simulink model "SeatMdSwtchArbt"  (R2018b)
settings: Solver=FixedStepDiscrete  StartTime=0.0  StopTime=10.0  FixedStep=0.01  RelTol=1e-3
undefined symbols (not defined in the file or in its folder): PosRclRspStat1
libraries: SeatMdSwtchArbt_Lib x35
(part 1 of 2)
settings Model: Creator=su3dcu  LastModifiedBy=su3dcu
settings DataIOCC: SaveFormat=StructureWithTime  ReturnWorkspaceOutputs=on
settings OptimizationCC: DefaultParameterBehavior=Inlined  EnhancedBackFolding=on  PassReuseOutputArgsAs=Individual arguments  ZeroExternalMemoryAtStartup=off  ZeroInternalMemoryAtStartup=off  OptimizeBlockOrder=speed  DifferentSizesBufferReuse=on  OptimizationCustomize=off
settings DebuggingCC: ParameterTunabilityLossMsg=error
settings HardwareCC: ProdBitPerPointer=32  ProdBitPerSizeT=32  ProdBitPerPtrDiffT=32  ProdLargestAtomicFloat=None  ProdWordSize=32  ProdHWDeviceType=Renesas->RH850
settings ModelReferenceCC: ModelReferenceNumInstancesAllowed=Single
settings SFSimCC: SimCustomHeaderCode="#include\"Rte_Type.h\""  MATLABDynamicMemAlloc=off
settings RTWCC: SystemTargetFile=autosar.tlc  GenCodeOnly=on  TemplateMakefile=ert_default_tmf  Description=AUTOSAR  GenerateReport=on  IncludeHyperlinkInReport=on  LaunchReport=on  CodeExecutionProfiling=on  GenerateTraceInfo=on  GenerateTraceReport=on  GenerateTraceReportSl=on  GenerateTraceReportSf=on  GenerateTraceReportEml=on  GenerateCodeMetricsReport=on
settings CodeAppCC: ForceParamTrailComments=on  IgnoreCustomStorageClasses=off  MaxIdLength=63  OperatorAnnotations=on  SimulinkDataObjDesc=on  SFDataObjDesc=on  InsertBlockDesc=on
settings STFCustomTargetCC: TargetLangStandard=C99 (ISO)  MultiwordLength=256  ParMdlRefBuildCompliant=on  CompOptLevelCompliant=on  IncludeMdlTerminateFcn=off  CombineOutputUpdateFcns=on  SuppressErrorStatus=on  ERTCustomFileBanners=on  SupportAbsoluteTime=off  PurelyIntegerCode=on  SupportNonFinite=off  SupportComplex=off  SupportContinuousTime=off  SupportNonInlinedSFcns=off  RemoveResetFunc=on  MATLABClassNameForMDSCustomization=Simulink.SoftwareTarget.ERTCustomization  AutosarCompliant=on  UseToolchainInfoCompliant=on  LookupTableObjectStructAxisOrder=2,1,3,4,...  LUTObjectStructOrderEvenSpacing=Size,Table,Breakpoints  SystemTargetFile=autosar.tlc
settings ERTTargetCC: TargetLangStandard=C99 (ISO)  ConcurrentExecutionCompliant=off  IncludeMdlTerminateFcn=off  SuppressErrorStatus=on  SupportAbsoluteTime=off  PurelyIntegerCode=on  SupportNonFinite=off  SupportComplex=off  ModelStepFunctionPrototypeControlCompliant=off  CPPClassGenCompliant=off  AutosarCompliant=on  LookupTableObjectStructAxisOrder=2,1,3,4,...  LUTObjectStructOrderEvenSpacing=Size,Table,Breakpoints  InlinedParameterPlacement=NonHierarchical  ERTCustomFileTemplate=example_file_process.tlc  ERTFilePackagingFormat=Compact
settings ConfigComp: DVTestSuiteOptimization=CombinedObjectives (Nonlinear Extended)  DVDetectActiveLogic=on  DVDetectOutOfBounds=on

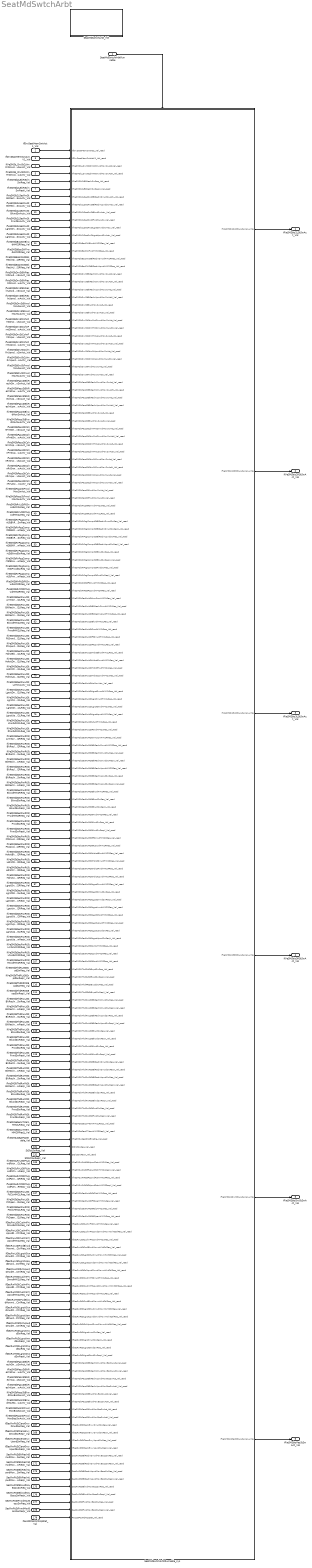
== system SeatMdSwtchArbt ==
  SeatMdSwtchArbtRunnable : Inport  SampleTime=0.01  OutputFunctionCall=on
  IfDrvSeatMemSwtAct1_Val : Inport  Port=2  OutDataTypeStr=Enum: TeSMS_e_DrvStMemSwAct  PortDimensions=1
  IfDrvSeatMemSwtActV1_Val : Inport  Port=3  OutDataTypeStr=Enum: TeSMS_e_DrvStMemSwActV  PortDimensions=1
  IfVeSMSb_DrvStCshnRrDnwdMovSwAct_Val : Inport  Port=4  OutDataTypeStr=boolean  PortDimensions=1
  IfVeSMSb_DrvStCshnRrDnwdMovSwActV_Val : Inport  Port=5  OutDataTypeStr=boolean  PortDimensions=1
  IfVeSMSb2LBkReclnSwReq_Val : Inport  Port=6  OutDataTypeStr=uint8  PortDimensions=1
  IfVeSMSb2LBkReclnSwReqV_Val : Inport  Port=7  OutDataTypeStr=boolean  PortDimensions=1
  IfVeSMSb2LSecRwStBkReclnDnwdSwActv_Val : Inport  Port=8  OutDataTypeStr=boolean  PortDimensions=1
  IfVeSMSb2LSecRwStBkReclnUpwdSwActv_Val : Inport  Port=9  OutDataTypeStr=boolean  PortDimensions=1
  IfVeSMSb2LSecRwStBkwdSwActv_Val : Inport  Port=10  OutDataTypeStr=boolean  PortDimensions=1
  IfVeSMSb2LSecRwStFrwdSwActv_Val : Inport  Port=11  OutDataTypeStr=boolean  PortDimensions=1
  IfVeSMSb2LSecRwStLgrstDnwdSwActv_Val : Inport  Port=12  OutDataTypeStr=boolean  PortDimensions=1
  IfVeSMSb2LSecRwStLgrstUpwdSwActv_Val : Inport  Port=13  OutDataTypeStr=boolean  PortDimensions=1
  IfVeSMSbBosSWBkwdHMI2RReq_Val : Inport  Port=14  OutDataTypeStr=boolean  PortDimensions=1
  IfVeSMSbBosSWFrwdHMI2RReq_Val : Inport  Port=15  OutDataTypeStr=boolean  PortDimensions=1
  IfVeSMSbBosSWStBkReclnDnwdHMI2RReq_Val : Inport  Port=16  OutDataTypeStr=boolean  PortDimensions=1
  IfVeSMSbBosSWStBkReclnUpwdHMI2RReq_Val : Inport  Port=17  OutDataTypeStr=boolean  PortDimensions=1
  IfVeSMSbDrvStBkReclnDnwdMovSwAct_Val : Inport  Port=18  OutDataTypeStr=boolean  PortDimensions=1
  IfVeSMSbDrvStBkReclnDnwdMovSwActV_Val : Inport  Port=19  OutDataTypeStr=boolean  PortDimensions=1
  IfVeSMSbDrvStBkReclnUpwdMovSwAct_Val : Inport  Port=20  OutDataTypeStr=boolean  PortDimensions=1
  IfVeSMSbDrvStBkReclnUpwdMovSwActV_Val : Inport  Port=21  OutDataTypeStr=boolean  PortDimensions=1
  IfVeSMSbDrvStBkwdMovSwAct_Val : Inport  Port=22  OutDataTypeStr=boolean  PortDimensions=1
  IfVeSMSbDrvStBkwdMovSwActV_Val : Inport  Port=23  OutDataTypeStr=boolean  PortDimensions=1
  IfVeSMSbDrvStCshnFrntDnwdMovSwAct_Val : Inport  Port=24  OutDataTypeStr=boolean  PortDimensions=1
  IfVeSMSbDrvStCshnFrntDnwdMovSwActV_Val : Inport  Port=25  OutDataTypeStr=boolean  PortDimensions=1
  IfVeSMSbDrvStCshnFrntUpwdMovSwAct_Val : Inport  Port=26  OutDataTypeStr=boolean  PortDimensions=1
  IfVeSMSbDrvStCshnFrntUpwdMovSwActV_Val : Inport  Port=27  OutDataTypeStr=boolean  PortDimensions=1
  IfVeSMSbDrvStCshnRrUpwdMovSwAct_Val : Inport  Port=28  OutDataTypeStr=boolean  PortDimensions=1
  IfVeSMSbDrvStCshnRrUpwdMovSwActV_Val : Inport  Port=29  OutDataTypeStr=boolean  PortDimensions=1
  IfVeSMSbDrvStFrwdMovSwAct_Val : Inport  Port=30  OutDataTypeStr=boolean  PortDimensions=1
  IfVeSMSbDrvStFrwdMovSwActV_Val : Inport  Port=31  OutDataTypeStr=boolean  PortDimensions=1
  IfVeSMSbPassStBkReclnDnwdMovSwAct_Val : Inport  Port=32  OutDataTypeStr=boolean  PortDimensions=1
  IfVeSMSbPassStBkReclnDnwdMovSwActV_Val : Inport  Port=33  OutDataTypeStr=boolean  PortDimensions=1
  IfVeSMSbPassStBkReclnUpwdMovSwAct_Val : Inport  Port=34  OutDataTypeStr=boolean  PortDimensions=1
  IfVeSMSbPassStBkReclnUpwdMovSwActV_Val : Inport  Port=35  OutDataTypeStr=boolean  PortDimensions=1
  IfVeSMSbPassStBkwdMovSwAct_Val : Inport  Port=36  OutDataTypeStr=boolean  PortDimensions=1
  IfVeSMSbPassStBkwdMovSwActV_Val : Inport  Port=37  OutDataTypeStr=boolean  PortDimensions=1
  IfVeSMSbPassStCshnFrntDnwdMovSwAct_Val : Inport  Port=38  OutDataTypeStr=boolean  PortDimensions=1
  IfVeSMSbPassStCshnFrntDnwdMovSwActV_Val : Inport  Port=39  OutDataTypeStr=boolean  PortDimensions=1
  IfVeSMSbPassStCshnFrntUpwdMovSwAct_Val : Inport  Port=40  OutDataTypeStr=boolean  PortDimensions=1
  IfVeSMSbPassStCshnFrntUpwdMovSwActV_Val : Inport  Port=41  OutDataTypeStr=boolean  PortDimensions=1
  IfVeSMSbPassStCshnRrDnwdMovSwAct_Val : Inport  Port=42  OutDataTypeStr=boolean  PortDimensions=1
  IfVeSMSbPassStCshnRrDnwdMovSwActV_Val : Inport  Port=43  OutDataTypeStr=boolean  PortDimensions=1
  IfVeSMSbPassStCshnRrUpwdMovSwAct_Val : Inport  Port=44  OutDataTypeStr=boolean  PortDimensions=1
  IfVeSMSbPassStCshnRrUpwdMovSwActV_Val : Inport  Port=45  OutDataTypeStr=boolean  PortDimensions=1
  IfVeSMSbPassStFrwdMovSwAct_Val : Inport  Port=46  OutDataTypeStr=boolean  PortDimensions=1
  IfVeSMSbPassStFrwdMovSwActV_Val : Inport  Port=47  OutDataTypeStr=boolean  PortDimensions=1
  IfVeSMSbRrLtStFtDnwdHMI2LReq_Val : Inport  Port=48  OutDataTypeStr=boolean  PortDimensions=1
  IfVeSMSbRrLtStFtUpwdHMI2LReq_Val : Inport  Port=49  OutDataTypeStr=boolean  PortDimensions=1
  IfVeSMSbRrPsgComprtStBkReclnDnwdSwReq_Val : Inport  Port=50  OutDataTypeStr=boolean  PortDimensions=1
  IfVeSMSbRrPsgComprtStBkReclnDnwdSwReqV_Val : Inport  Port=51  OutDataTypeStr=boolean  PortDimensions=1
  IfVeSMSbRrPsgComprtStBkReclnUpwdSwReq_Val : Inport  Port=52  OutDataTypeStr=boolean  PortDimensions=1
  IfVeSMSbRrPsgComprtStBkReclnUpwdSwReqV_Val : Inport  Port=53  OutDataTypeStr=boolean  PortDimensions=1
  IfVeSMSbRrPsgComprtStBkwdSwReq_Val : Inport  Port=54  OutDataTypeStr=boolean  PortDimensions=1
  IfVeSMSbRrPsgComprtStBkwdSwReqV_Val : Inport  Port=55  OutDataTypeStr=boolean  PortDimensions=1
  IfVeSMSbRrPsgComprtStFrwdSwReq_Val : Inport  Port=56  OutDataTypeStr=boolean  PortDimensions=1
  IfVeSMSbRrPsgComprtStFrwdSwReqV_Val : Inport  Port=57  OutDataTypeStr=boolean  PortDimensions=1
  IfVeSMSbRrRtStFtDnwdHMI2RReq_Val : Inport  Port=58  OutDataTypeStr=boolean  PortDimensions=1
  IfVeSMSbRrRtStFtUpwdHMI2RReq_Val : Inport  Port=59  OutDataTypeStr=boolean  PortDimensions=1
  IfVeSMSbSecRwLtStArmScrnHMI2LReq_Val : Inport  Port=60  OutDataTypeStr=boolean  PortDimensions=1
  IfVeSMSbSecRwLtStBkReclnDnwdHMI2LReq_Val : Inport  Port=61  OutDataTypeStr=boolean  PortDimensions=1
  IfVeSMSbSecRwLtStBkReclnUpwdHMI2LReq_Val : Inport  Port=62  OutDataTypeStr=boolean  PortDimensions=1
  IfVeSMSbSecRwLtStBkwdHMI2LReq_Val : Inport  Port=63  OutDataTypeStr=boolean  PortDimensions=1
  IfVeSMSbSecRwLtStFrwdHMI2LReq_Val : Inport  Port=64  OutDataTypeStr=boolean  PortDimensions=1
  IfVeSMSbSecRwLtStFtDnwdHMI2LReq_Val : Inport  Port=65  OutDataTypeStr=boolean  PortDimensions=1
  IfVeSMSbSecRwLtStFtUpwdHMI2LReq_Val : Inport  Port=66  OutDataTypeStr=boolean  PortDimensions=1
  IfVeSMSbSecRwLtStHdrstBkwdHMI2LReq_Val : Inport  Port=67  OutDataTypeStr=boolean  PortDimensions=1
  IfVeSMSbSecRwLtStHdrstDnwdHMI2LReq_Val : Inport  Port=68  OutDataTypeStr=boolean  PortDimensions=1
  IfVeSMSbSecRwLtStHdrstFrwdHMI2LReq_Val : Inport  Port=69  OutDataTypeStr=boolean  PortDimensions=1
  IfVeSMSbSecRwLtStHdrstUpwdHMI2LReq_Val : Inport  Port=70  OutDataTypeStr=boolean  PortDimensions=1
  IfVeSMSbSecRwLtStLcMovActv_Val : Inport  Port=71  OutDataTypeStr=boolean  PortDimensions=1
  IfVeSMSbSecRwLtStLgrstDnwdHMI2LReq_Val : Inport  Port=72  OutDataTypeStr=boolean  PortDimensions=1
  IfVeSMSbSecRwLtStLgrstInwdHMI2LReq_Val : Inport  Port=73  OutDataTypeStr=boolean  PortDimensions=1
  IfVeSMSbSecRwLtStLgrstOtwdHMI2LReq_Val : Inport  Port=74  OutDataTypeStr=boolean  PortDimensions=1
  IfVeSMSbSecRwLtStLgrstUpwdHMI2LReq_Val : Inport  Port=75  OutDataTypeStr=boolean  PortDimensions=1
  IfVeSMSbSecRwLtStLtwdHMI2LReq_Val : Inport  Port=76  OutDataTypeStr=boolean  PortDimensions=1
  IfVeSMSbSecRwLtStRtwdHMI2LReq_Val : Inport  Port=77  OutDataTypeStr=boolean  PortDimensions=1
  IfVeSMSbSecRwRtStArmScrnHMI2RReq_Val : Inport  Port=78  OutDataTypeStr=boolean  PortDimensions=1
  IfVeSMSbSecRwRtStBkReclnDnwdHMI2RReq_Val : Inport  Port=79  OutDataTypeStr=boolean  PortDimensions=1
  IfVeSMSbSecRwRtStBkReclnDnwdSwReq_Val : Inport  Port=80  OutDataTypeStr=boolean  PortDimensions=1
  IfVeSMSbSecRwRtStBkReclnDnwdSwReqV_Val : Inport  Port=81  OutDataTypeStr=boolean  PortDimensions=1
  IfVeSMSbSecRwRtStBkReclnUpwdHMI2RReq_Val : Inport  Port=82  OutDataTypeStr=boolean  PortDimensions=1
  IfVeSMSbSecRwRtStBkReclnUpwdSwReq_Val : Inport  Port=83  OutDataTypeStr=boolean  PortDimensions=1
  IfVeSMSbSecRwRtStBkReclnUpwdSwReqV_Val : Inport  Port=84  OutDataTypeStr=boolean  PortDimensions=1
  IfVeSMSbSecRwRtStBkwdHMI2RReq_Val : Inport  Port=85  OutDataTypeStr=boolean  PortDimensions=1
  IfVeSMSbSecRwRtStBkwdSwReq_Val : Inport  Port=86  OutDataTypeStr=boolean  PortDimensions=1
  IfVeSMSbSecRwRtStBkwdSwReqV_Val : Inport  Port=87  OutDataTypeStr=boolean  PortDimensions=1
  IfVeSMSbSecRwRtStFrwdHMI2RReq_Val : Inport  Port=88  OutDataTypeStr=boolean  PortDimensions=1
  IfVeSMSbSecRwRtStFrwdSwReq_Val : Inport  Port=89  OutDataTypeStr=boolean  PortDimensions=1
  IfVeSMSbSecRwRtStFrwdSwReqV_Val : Inport  Port=90  OutDataTypeStr=boolean  PortDimensions=1
  IfVeSMSbSecRwRtStFtDnwdHMI2RReq_Val : Inport  Port=91  OutDataTypeStr=boolean  PortDimensions=1
  IfVeSMSbSecRwRtStFtUpwdHMI2RReq_Val : Inport  Port=92  OutDataTypeStr=boolean  PortDimensions=1
  IfVeSMSbSecRwRtStHdrstBkwdHMI2RReq_Val : Inport  Port=93  OutDataTypeStr=boolean  PortDimensions=1
  IfVeSMSbSecRwRtStHdrstDnwdHMI2RReq_Val : Inport  Port=94  OutDataTypeStr=boolean  PortDimensions=1
  IfVeSMSbSecRwRtStHdrstFrwdHMI2RReq_Val : Inport  Port=95  OutDataTypeStr=boolean  PortDimensions=1
  IfVeSMSbSecRwRtStHdrstUpwdHMI2RReq_Val : Inport  Port=96  OutDataTypeStr=boolean  PortDimensions=1
  IfVeSMSbSecRwRtStLgrstDnwdHMI2RReq_Val : Inport  Port=97  OutDataTypeStr=boolean  PortDimensions=1
  IfVeSMSbSecRwRtStLgrstDnwdSwReq_Val : Inport  Port=98  OutDataTypeStr=boolean  PortDimensions=1
  IfVeSMSbSecRwRtStLgrstDnwdSwReqV_Val : Inport  Port=99  OutDataTypeStr=boolean  PortDimensions=1
  IfVeSMSbSecRwRtStLgrstInwdHMI2RReq_Val : Inport  Port=100  OutDataTypeStr=boolean  PortDimensions=1
  IfVeSMSbSecRwRtStLgrstOtwdHMI2RReq_Val : Inport  Port=101  OutDataTypeStr=boolean  PortDimensions=1
  IfVeSMSbSecRwRtStLgrstUpwdHMI2RReq_Val : Inport  Port=102  OutDataTypeStr=boolean  PortDimensions=1
  IfVeSMSbSecRwRtStLgrstUpwdSwReq_Val : Inport  Port=103  OutDataTypeStr=boolean  PortDimensions=1
  IfVeSMSbSecRwRtStLgrstUpwdSwReqV_Val : Inport  Port=104  OutDataTypeStr=boolean  PortDimensions=1
  IfVeSMSbSecRwRtStLmbrHMI2RReq_Val : Inport  Port=105  OutDataTypeStr=Enum: SeatLmbrSwtchType  PortDimensions=1
  IfVeSMSbSecRwRtStLtwdHMI2RReq_Val : Inport  Port=106  OutDataTypeStr=boolean  PortDimensions=1
  IfVeSMSbSecRwRtStRtwdHMI2RReq_Val : Inport  Port=107  OutDataTypeStr=boolean  PortDimensions=1
  IfVeSMSbThdRLtStExpdSwReq_Val : Inport  Port=108  OutDataTypeStr=boolean  PortDimensions=1
  IfVeSMSbThdRLtStExpdSwReqV_Val : Inport  Port=109  OutDataTypeStr=boolean  PortDimensions=1
  IfVeSMSbThdRRtStExpdSwReq_Val : Inport  Port=110  OutDataTypeStr=boolean  PortDimensions=1
  IfVeSMSbThdRRtStExpdSwReqV_Val : Inport  Port=111  OutDataTypeStr=boolean  PortDimensions=1
  IfVeSMSbThdRwLtStBkReclnDnwdSwReq_Val : Inport  Port=112  OutDataTypeStr=boolean  PortDimensions=1
  IfVeSMSbThdRwLtStBkReclnDnwdSwReqV_Val : Inport  Port=113  OutDataTypeStr=boolean  PortDimensions=1
  IfVeSMSbThdRwLtStBkReclnUpwdSwReq_Val : Inport  Port=114  OutDataTypeStr=boolean  PortDimensions=1
  IfVeSMSbThdRwLtStBkReclnUpwdSwReqV_Val : Inport  Port=115  OutDataTypeStr=boolean  PortDimensions=1
  IfVeSMSbThdRwLtStBkwdSwReq_Val : Inport  Port=116  OutDataTypeStr=boolean  PortDimensions=1
  IfVeSMSbThdRwLtStBkwdSwReqV_Val : Inport  Port=117  OutDataTypeStr=boolean  PortDimensions=1
  IfVeSMSbThdRwLtStFrwdSwReq_Val : Inport  Port=118  OutDataTypeStr=boolean  PortDimensions=1
  IfVeSMSbThdRwLtStFrwdSwReqV_Val : Inport  Port=119  OutDataTypeStr=boolean  PortDimensions=1
  IfVeSMSbThdRwRtStBkReclnDnwdSwReq_Val : Inport  Port=120  OutDataTypeStr=boolean  PortDimensions=1
  IfVeSMSbThdRwRtStBkReclnDnwdSwReqV_Val : Inport  Port=121  OutDataTypeStr=boolean  PortDimensions=1
  IfVeSMSbThdRwRtStBkReclnUpwdSwReq_Val : Inport  Port=122  OutDataTypeStr=boolean  PortDimensions=1
  IfVeSMSbThdRwRtStBkReclnUpwdSwReqV_Val : Inport  Port=123  OutDataTypeStr=boolean  PortDimensions=1
  IfVeSMSbThdRwRtStBkwdSwReq_Val : Inport  Port=124  OutDataTypeStr=boolean  PortDimensions=1
  IfVeSMSbThdRwRtStBkwdSwReqV_Val : Inport  Port=125  OutDataTypeStr=boolean  PortDimensions=1
  IfVeSMSbThdRwRtStFrwdSwReq_Val : Inport  Port=126  OutDataTypeStr=boolean  PortDimensions=1
  IfVeSMSbThdRwRtStFrwdSwReqV_Val : Inport  Port=127  OutDataTypeStr=boolean  PortDimensions=1
  IfVeSMSeSecLTMemHMI2LReq1_Val : Inport  Port=128  OutDataTypeStr=Enum: TeSMS_e_SecLTSeatMemHMIReq  PortDimensions=1
  IfVeSMSeSecLTMemHMI2RReq1_Val : Inport  Port=129  OutDataTypeStr=Enum: TeSMS_e_SecLTSeatMemHMIReq  PortDimensions=1
  IfVeSMSuSeatPosEnable_Val : Inport  Port=130  OutDataTypeStr=uint8  PortDimensions=1
  StSlctSwReq_Val : Inport  Port=131  OutDataTypeStr=Enum: LugSelectSw1  PortDimensions=1
  StSlctSwReqV_Val : Inport  Port=132  OutDataTypeStr=boolean  PortDimensions=1
  IfVeSMSuRrLtStFtUpwdPstnHMI2LReq_Val : Inport  Port=133  OutDataTypeStr=uint16  PortDimensions=1
  IfVeSMSuRrLtStFtUpwdPstnHMI2LReqV_Val : Inport  Port=134  OutDataTypeStr=boolean  PortDimensions=1
  IfVeSMSuRrRtStFtUpwdPstnHMI2RReq_Val : Inport  Port=135  OutDataTypeStr=uint16  PortDimensions=1
  IfVeSMSuRrRtStFtUpwdPstnHMI2RReqV_Val : Inport  Port=136  OutDataTypeStr=boolean  PortDimensions=1
  IfVeSMSbSecRwLtStFtClsHMI2LReq_Val : Inport  Port=137  OutDataTypeStr=boolean  PortDimensions=1
  IfVeSMSbSecRwLtStFtOpenHMI2LReq_Val : Inport  Port=138  OutDataTypeStr=boolean  PortDimensions=1
  IfVeSMSbSecRwRtStFtClsHMI2LReq_Val : Inport  Port=139  OutDataTypeStr=boolean  PortDimensions=1
  IfVeSMSbSecRwRtStFtOpenHMI2LReq_Val : Inport  Port=140  OutDataTypeStr=boolean  PortDimensions=1
  IfSecRwLtStCushnFrtDnwdHMI2LReq_Val : Inport  Port=141  OutDataTypeStr=boolean  PortDimensions=1
  IfSecRwLtStCushnFrtUpwdDnwdMovmtVirtCtrlReq_Val : Inport  Port=142  OutDataTypeStr=Enum: UpwdDnwdMovmtVirtCtrlReq  PortDimensions=1
  IfSecRwLtStCushnFrtUpwdHMI2LReq_Val : Inport  Port=143  OutDataTypeStr=boolean  PortDimensions=1
  IfSecRwLtStFwdBkwdMovmtVirtCtrlReq_Val : Inport  Port=144  OutDataTypeStr=Enum: FwdBkwdMovmtVirtCtrlReq  PortDimensions=1
  IfSecRwLtStLgrstOtwdInwdMovmtVirtCtrlReq_Val : Inport  Port=145  OutDataTypeStr=Enum: OtwdInwdMovmtVirtCtrlReq  PortDimensions=1
  IfSecRwLtStLgrstUpwdDnwdMovmtVirtCtrlReq_Val : Inport  Port=146  OutDataTypeStr=Enum: UpwdDnwdMovmtVirtCtrlReq  PortDimensions=1
  IfSecRwLtStRclUpwdDnwdMovmtVirtCtrlReq_Val : Inport  Port=147  OutDataTypeStr=Enum: UpwdDnwdMovmtVirtCtrlReq  PortDimensions=1
  IfSecRwRtStCushnFrtDnwdHMI2LReq_Val : Inport  Port=148  OutDataTypeStr=boolean  PortDimensions=1
  IfSecRwRtStCushnFrtUpwdDnwdMovmtVirtCtrlReq_Val : Inport  Port=149  OutDataTypeStr=Enum: UpwdDnwdMovmtVirtCtrlReq  PortDimensions=1
  IfSecRwRtStCushnFrtUpwdHMI2LReq_Val : Inport  Port=150  OutDataTypeStr=boolean  PortDimensions=1
  IfSecRwRtStFwdBkwdMovmtVirtCtrlReq_Val : Inport  Port=151  OutDataTypeStr=Enum: FwdBkwdMovmtVirtCtrlReq  PortDimensions=1
  IfSecRwRtStLgrstOtwdInwdMovmtVirtCtrlReq_Val : Inport  Port=152  OutDataTypeStr=Enum: OtwdInwdMovmtVirtCtrlReq  PortDimensions=1
  IfSecRwRtStLgrstUpwdDnwdMovmtVirtCtrlReq_Val : Inport  Port=153  OutDataTypeStr=Enum: UpwdDnwdMovmtVirtCtrlReq  PortDimensions=1
  IfSecRwRtStRclUpwdDnwdMovmtVirtCtrlReq_Val : Inport  Port=154  OutDataTypeStr=Enum: UpwdDnwdMovmtVirtCtrlReq  PortDimensions=1
  IfSecRwRtStLgrstInwdSwReq_Val : Inport  Port=155  OutDataTypeStr=boolean  PortDimensions=1
  IfSecRwRtStLgrstInwdSwReqV_Val : Inport  Port=156  OutDataTypeStr=boolean  PortDimensions=1
  IfSecRwRtStLgrstOtwdSwReq_Val : Inport  Port=157  OutDataTypeStr=boolean  PortDimensions=1
  IfSecRwRtStLgrstOtwdSwReqV_Val : Inport  Port=158  OutDataTypeStr=boolean  PortDimensions=1
  IfVeSMSbPassStBkReclnDnwdMovBosSwAct_Val : Inport  Port=159  OutDataTypeStr=boolean  PortDimensions=1
  IfVeSMSbPassStBkReclnDnwdMovBosSwActV_Val : Inport  Port=160  OutDataTypeStr=boolean  PortDimensions=1
  IfVeSMSbPassStBkReclnUpwdMovBosSwAct_Val : Inport  Port=161  OutDataTypeStr=boolean  PortDimensions=1
  IfVeSMSbPassStBkReclnUpwdMovBosSwActV_Val : Inport  Port=162  OutDataTypeStr=boolean  PortDimensions=1
  IfVeSMSbPassStBkwdMovBosSwAct_Val : Inport  Port=163  OutDataTypeStr=boolean  PortDimensions=1
  IfVeSMSbPassStBkwdMovBosSwActV_Val : Inport  Port=164  OutDataTypeStr=boolean  PortDimensions=1
  IfVeSMSbPassStFrwdMovBosSwAct_Val : Inport  Port=165  OutDataTypeStr=boolean  PortDimensions=1
  IfVeSMSbPassStFrwdMovBosSwActV_Val : Inport  Port=166  OutDataTypeStr=boolean  PortDimensions=1
  IfSecRwRtStZeroGrvyDnwdSwReq_Val : Inport  Port=167  OutDataTypeStr=boolean  PortDimensions=1
  IfSecRwRtStZeroGrvyDnwdSwReqV_Val : Inport  Port=168  OutDataTypeStr=boolean  PortDimensions=1
  IfSecRwRtStZeroGrvyUpwdSwReq_Val : Inport  Port=169  OutDataTypeStr=boolean  PortDimensions=1
  IfSecRwRtStZeroGrvyUpwdSwReqV_Val : Inport  Port=170  OutDataTypeStr=boolean  PortDimensions=1
  SecRwRtStBkReclnDnwdMovBossSwReq_Val : Inport  Port=171  OutDataTypeStr=boolean  PortDimensions=1
  SecRwRtStBkReclnDnwdMovBossSwReqV_Val : Inport  Port=172  OutDataTypeStr=boolean  PortDimensions=1
  SecRwRtStBkReclnUpwdMovBossSwReq_Val : Inport  Port=173  OutDataTypeStr=boolean  PortDimensions=1
  SecRwRtStBkReclnUpwdMovBossSwReqV_Val : Inport  Port=174  OutDataTypeStr=boolean  PortDimensions=1
  SecRwRtStBkwdMovBossSwReq_Val : Inport  Port=175  OutDataTypeStr=boolean  PortDimensions=1
  SecRwRtStBkwdMovBossSwReqV_Val : Inport  Port=176  OutDataTypeStr=boolean  PortDimensions=1
  SecRwRtStFrwdMovBossSwReq_Val : Inport  Port=177  OutDataTypeStr=boolean  PortDimensions=1
  SecRwRtStFrwdMovBossSwReqV_Val : Inport  Port=178  OutDataTypeStr=boolean  PortDimensions=1
  PassStPosRclRspStat_Val : Inport  Port=179  OutDataTypeStr=Enum: PosRclRspStat1  PortDimensions=1
  SeatMdSwtchArbtRunnable_sys : Subsystem
  SeatMdSwtchArbt_Init : Subsystem
  IfVeSMSbIs2LStSwAct_Val : Outport  OutDataTypeStr=boolean  PortDimensions=1
  IfVeSMSbIs2RStSwAct_Val : Outport  Port=2  OutDataTypeStr=boolean  PortDimensions=1
  IfVeSMSbIs3LStSwAct_Val : Outport  Port=3  OutDataTypeStr=boolean  PortDimensions=1
  IfVeSMSbIs3RStSwAct_Val : Outport  Port=4  OutDataTypeStr=boolean  PortDimensions=1
  IfVeSMSbIsDrvStSwAct_Val : Outport  Port=5  OutDataTypeStr=boolean  PortDimensions=1
  IfVeSMSbIsPasStSwAct_Val : Outport  Port=6  OutDataTypeStr=boolean  PortDimensions=1
  wires:
  IfDrvSeatMemSwtAct1_Val/1 -> SeatMdSwtchArbtRunnable_sys/1(IfDrvSeatMemSwtAct1_Val_read)
  IfDrvSeatMemSwtActV1_Val/1 -> SeatMdSwtchArbtRunnable_sys/2(IfDrvSeatMemSwtActV1_Val_read)
  IfVeSMSb_DrvStCshnRrDnwdMovSwAct_Val/1 -> SeatMdSwtchArbtRunnable_sys/3(IfVeSMSb_DrvStCshnRrDnwdMovSwAct_Val_read)
  IfVeSMSb_DrvStCshnRrDnwdMovSwActV_Val/1 -> SeatMdSwtchArbtRunnable_sys/4(IfVeSMSb_DrvStCshnRrDnwdMovSwActV_Val_read)
  IfVeSMSb2LBkReclnSwReq_Val/1 -> SeatMdSwtchArbtRunnable_sys/5(IfVeSMSb2LBkReclnSwReq_Val_read)
  IfVeSMSb2LBkReclnSwReqV_Val/1 -> SeatMdSwtchArbtRunnable_sys/6(IfVeSMSb2LBkReclnSwReqV_Val_read)
  IfVeSMSb2LSecRwStBkReclnDnwdSwActv_Val/1 -> SeatMdSwtchArbtRunnable_sys/7(IfVeSMSb2LSecRwStBkReclnDnwdSwActv_Val_read)
  IfVeSMSb2LSecRwStBkReclnUpwdSwActv_Val/1 -> SeatMdSwtchArbtRunnable_sys/8(IfVeSMSb2LSecRwStBkReclnUpwdSwActv_Val_read)
  IfVeSMSb2LSecRwStBkwdSwActv_Val/1 -> SeatMdSwtchArbtRunnable_sys/9(IfVeSMSb2LSecRwStBkwdSwActv_Val_read)
  IfVeSMSb2LSecRwStFrwdSwActv_Val/1 -> SeatMdSwtchArbtRunnable_sys/10(IfVeSMSb2LSecRwStFrwdSwActv_Val_read)
  IfVeSMSb2LSecRwStLgrstDnwdSwActv_Val/1 -> SeatMdSwtchArbtRunnable_sys/11(IfVeSMSb2LSecRwStLgrstDnwdSwActv_Val_read)
  IfVeSMSb2LSecRwStLgrstUpwdSwActv_Val/1 -> SeatMdSwtchArbtRunnable_sys/12(IfVeSMSb2LSecRwStLgrstUpwdSwActv_Val_read)
  IfVeSMSbBosSWBkwdHMI2RReq_Val/1 -> SeatMdSwtchArbtRunnable_sys/13(IfVeSMSbBosSWBkwdHMI2RReq_Val_read)
  IfVeSMSbBosSWFrwdHMI2RReq_Val/1 -> SeatMdSwtchArbtRunnable_sys/14(IfVeSMSbBosSWFrwdHMI2RReq_Val_read)
  IfVeSMSbBosSWStBkReclnDnwdHMI2RReq_Val/1 -> SeatMdSwtchArbtRunnable_sys/15(IfVeSMSbBosSWStBkReclnDnwdHMI2RReq_Val_read)
  IfVeSMSbBosSWStBkReclnUpwdHMI2RReq_Val/1 -> SeatMdSwtchArbtRunnable_sys/16(IfVeSMSbBosSWStBkReclnUpwdHMI2RReq_Val_read)
  IfVeSMSbDrvStBkReclnDnwdMovSwAct_Val/1 -> SeatMdSwtchArbtRunnable_sys/17(IfVeSMSbDrvStBkReclnDnwdMovSwAct_Val_read)
  IfVeSMSbDrvStBkReclnDnwdMovSwActV_Val/1 -> SeatMdSwtchArbtRunnable_sys/18(IfVeSMSbDrvStBkReclnDnwdMovSwActV_Val_read)
  IfVeSMSbDrvStBkReclnUpwdMovSwAct_Val/1 -> SeatMdSwtchArbtRunnable_sys/19(IfVeSMSbDrvStBkReclnUpwdMovSwAct_Val_read)
  IfVeSMSbDrvStBkReclnUpwdMovSwActV_Val/1 -> SeatMdSwtchArbtRunnable_sys/20(IfVeSMSbDrvStBkReclnUpwdMovSwActV_Val_read)
  IfVeSMSbDrvStBkwdMovSwAct_Val/1 -> SeatMdSwtchArbtRunnable_sys/21(IfVeSMSbDrvStBkwdMovSwAct_Val_read)
  IfVeSMSbDrvStBkwdMovSwActV_Val/1 -> SeatMdSwtchArbtRunnable_sys/22(IfVeSMSbDrvStBkwdMovSwActV_Val_read)
  IfVeSMSbDrvStCshnFrntDnwdMovSwAct_Val/1 -> SeatMdSwtchArbtRunnable_sys/23(IfVeSMSbDrvStCshnFrntDnwdMovSwAct_Val_read)
  IfVeSMSbDrvStCshnFrntDnwdMovSwActV_Val/1 -> SeatMdSwtchArbtRunnable_sys/24(IfVeSMSbDrvStCshnFrntDnwdMovSwActV_Val_read)
  IfVeSMSbDrvStCshnFrntUpwdMovSwAct_Val/1 -> SeatMdSwtchArbtRunnable_sys/25(IfVeSMSbDrvStCshnFrntUpwdMovSwAct_Val_read)
  IfVeSMSbDrvStCshnFrntUpwdMovSwActV_Val/1 -> SeatMdSwtchArbtRunnable_sys/26(IfVeSMSbDrvStCshnFrntUpwdMovSwActV_Val_read)
  IfVeSMSbDrvStCshnRrUpwdMovSwAct_Val/1 -> SeatMdSwtchArbtRunnable_sys/27(IfVeSMSbDrvStCshnRrUpwdMovSwAct_Val_read)
  IfVeSMSbDrvStCshnRrUpwdMovSwActV_Val/1 -> SeatMdSwtchArbtRunnable_sys/28(IfVeSMSbDrvStCshnRrUpwdMovSwActV_Val_read)
  IfVeSMSbDrvStFrwdMovSwAct_Val/1 -> SeatMdSwtchArbtRunnable_sys/29(IfVeSMSbDrvStFrwdMovSwAct_Val_read)
  IfVeSMSbDrvStFrwdMovSwActV_Val/1 -> SeatMdSwtchArbtRunnable_sys/30(IfVeSMSbDrvStFrwdMovSwActV_Val_read)
  IfVeSMSbPassStBkReclnDnwdMovSwAct_Val/1 -> SeatMdSwtchArbtRunnable_sys/31(IfVeSMSbPassStBkReclnDnwdMovSwAct_Val_read)
  IfVeSMSbPassStBkReclnDnwdMovSwActV_Val/1 -> SeatMdSwtchArbtRunnable_sys/32(IfVeSMSbPassStBkReclnDnwdMovSwActV_Val_read)
  IfVeSMSbPassStBkReclnUpwdMovSwAct_Val/1 -> SeatMdSwtchArbtRunnable_sys/33(IfVeSMSbPassStBkReclnUpwdMovSwAct_Val_read)
  IfVeSMSbPassStBkReclnUpwdMovSwActV_Val/1 -> SeatMdSwtchArbtRunnable_sys/34(IfVeSMSbPassStBkReclnUpwdMovSwActV_Val_read)
  IfVeSMSbPassStBkwdMovSwAct_Val/1 -> SeatMdSwtchArbtRunnable_sys/35(IfVeSMSbPassStBkwdMovSwAct_Val_read)
  IfVeSMSbPassStBkwdMovSwActV_Val/1 -> SeatMdSwtchArbtRunnable_sys/36(IfVeSMSbPassStBkwdMovSwActV_Val_read)
  IfVeSMSbPassStCshnFrntDnwdMovSwAct_Val/1 -> SeatMdSwtchArbtRunnable_sys/37(IfVeSMSbPassStCshnFrntDnwdMovSwAct_Val_read)
  IfVeSMSbPassStCshnFrntDnwdMovSwActV_Val/1 -> SeatMdSwtchArbtRunnable_sys/38(IfVeSMSbPassStCshnFrntDnwdMovSwActV_Val_read)
  IfVeSMSbPassStCshnFrntUpwdMovSwAct_Val/1 -> SeatMdSwtchArbtRunnable_sys/39(IfVeSMSbPassStCshnFrntUpwdMovSwAct_Val_read)
  IfVeSMSbPassStCshnFrntUpwdMovSwActV_Val/1 -> SeatMdSwtchArbtRunnable_sys/40(IfVeSMSbPassStCshnFrntUpwdMovSwActV_Val_read)
  IfVeSMSbPassStCshnRrDnwdMovSwAct_Val/1 -> SeatMdSwtchArbtRunnable_sys/41(IfVeSMSbPassStCshnRrDnwdMovSwAct_Val_read)
  IfVeSMSbPassStCshnRrDnwdMovSwActV_Val/1 -> SeatMdSwtchArbtRunnable_sys/42(IfVeSMSbPassStCshnRrDnwdMovSwActV_Val_read)
  IfVeSMSbPassStCshnRrUpwdMovSwAct_Val/1 -> SeatMdSwtchArbtRunnable_sys/43(IfVeSMSbPassStCshnRrUpwdMovSwAct_Val_read)
  IfVeSMSbPassStCshnRrUpwdMovSwActV_Val/1 -> SeatMdSwtchArbtRunnable_sys/44(IfVeSMSbPassStCshnRrUpwdMovSwActV_Val_read)
  IfVeSMSbPassStFrwdMovSwAct_Val/1 -> SeatMdSwtchArbtRunnable_sys/45(IfVeSMSbPassStFrwdMovSwAct_Val_read)
  IfVeSMSbPassStFrwdMovSwActV_Val/1 -> SeatMdSwtchArbtRunnable_sys/46(IfVeSMSbPassStFrwdMovSwActV_Val_read)
  IfVeSMSbRrLtStFtDnwdHMI2LReq_Val/1 -> SeatMdSwtchArbtRunnable_sys/47(IfVeSMSbRrLtStFtDnwdHMI2LReq_Val_read)
  IfVeSMSbRrLtStFtUpwdHMI2LReq_Val/1 -> SeatMdSwtchArbtRunnable_sys/48(IfVeSMSbRrLtStFtUpwdHMI2LReq_Val_read)
  IfVeSMSbRrPsgComprtStBkReclnDnwdSwReq_Val/1 -> SeatMdSwtchArbtRunnable_sys/49(IfVeSMSbRrPsgComprtStBkReclnDnwdSwReq_Val_read)
  IfVeSMSbRrPsgComprtStBkReclnDnwdSwReqV_Val/1 -> SeatMdSwtchArbtRunnable_sys/50(IfVeSMSbRrPsgComprtStBkReclnDnwdSwReqV_Val_read)
  IfVeSMSbRrPsgComprtStBkReclnUpwdSwReq_Val/1 -> SeatMdSwtchArbtRunnable_sys/51(IfVeSMSbRrPsgComprtStBkReclnUpwdSwReq_Val_read)
  IfVeSMSbRrPsgComprtStBkReclnUpwdSwReqV_Val/1 -> SeatMdSwtchArbtRunnable_sys/52(IfVeSMSbRrPsgComprtStBkReclnUpwdSwReqV_Val_read)
  IfVeSMSbRrPsgComprtStBkwdSwReq_Val/1 -> SeatMdSwtchArbtRunnable_sys/53(IfVeSMSbRrPsgComprtStBkwdSwReq_Val_read)
  IfVeSMSbRrPsgComprtStBkwdSwReqV_Val/1 -> SeatMdSwtchArbtRunnable_sys/54(IfVeSMSbRrPsgComprtStBkwdSwReqV_Val_read)
  IfVeSMSbRrPsgComprtStFrwdSwReq_Val/1 -> SeatMdSwtchArbtRunnable_sys/55(IfVeSMSbRrPsgComprtStFrwdSwReq_Val_read)
  IfVeSMSbRrPsgComprtStFrwdSwReqV_Val/1 -> SeatMdSwtchArbtRunnable_sys/56(IfVeSMSbRrPsgComprtStFrwdSwReqV_Val_read)
  IfVeSMSbRrRtStFtDnwdHMI2RReq_Val/1 -> SeatMdSwtchArbtRunnable_sys/57(IfVeSMSbRrRtStFtDnwdHMI2RReq_Val_read)
  IfVeSMSbRrRtStFtUpwdHMI2RReq_Val/1 -> SeatMdSwtchArbtRunnable_sys/58(IfVeSMSbRrRtStFtUpwdHMI2RReq_Val_read)
  IfVeSMSbSecRwLtStArmScrnHMI2LReq_Val/1 -> SeatMdSwtchArbtRunnable_sys/59(IfVeSMSbSecRwLtStArmScrnHMI2LReq_Val_read)
  IfVeSMSbSecRwLtStBkReclnDnwdHMI2LReq_Val/1 -> SeatMdSwtchArbtRunnable_sys/60(IfVeSMSbSecRwLtStBkReclnDnwdHMI2LReq_Val_read)
  IfVeSMSbSecRwLtStBkReclnUpwdHMI2LReq_Val/1 -> SeatMdSwtchArbtRunnable_sys/61(IfVeSMSbSecRwLtStBkReclnUpwdHMI2LReq_Val_read)
  IfVeSMSbSecRwLtStBkwdHMI2LReq_Val/1 -> SeatMdSwtchArbtRunnable_sys/62(IfVeSMSbSecRwLtStBkwdHMI2LReq_Val_read)
  IfVeSMSbSecRwLtStFrwdHMI2LReq_Val/1 -> SeatMdSwtchArbtRunnable_sys/63(IfVeSMSbSecRwLtStFrwdHMI2LReq_Val_read)
  IfVeSMSbSecRwLtStFtDnwdHMI2LReq_Val/1 -> SeatMdSwtchArbtRunnable_sys/64(IfVeSMSbSecRwLtStFtDnwdHMI2LReq_Val_read)
  IfVeSMSbSecRwLtStFtUpwdHMI2LReq_Val/1 -> SeatMdSwtchArbtRunnable_sys/65(IfVeSMSbSecRwLtStFtUpwdHMI2LReq_Val_read)
  IfVeSMSbSecRwLtStHdrstBkwdHMI2LReq_Val/1 -> SeatMdSwtchArbtRunnable_sys/66(IfVeSMSbSecRwLtStHdrstBkwdHMI2LReq_Val_read)
  IfVeSMSbSecRwLtStHdrstDnwdHMI2LReq_Val/1 -> SeatMdSwtchArbtRunnable_sys/67(IfVeSMSbSecRwLtStHdrstDnwdHMI2LReq_Val_read)
  IfVeSMSbSecRwLtStHdrstFrwdHMI2LReq_Val/1 -> SeatMdSwtchArbtRunnable_sys/68(IfVeSMSbSecRwLtStHdrstFrwdHMI2LReq_Val_read)
  IfVeSMSbSecRwLtStHdrstUpwdHMI2LReq_Val/1 -> SeatMdSwtchArbtRunnable_sys/69(IfVeSMSbSecRwLtStHdrstUpwdHMI2LReq_Val_read)
  IfVeSMSbSecRwLtStLcMovActv_Val/1 -> SeatMdSwtchArbtRunnable_sys/70(IfVeSMSbSecRwLtStLcMovActv_Val_read)
  IfVeSMSbSecRwLtStLgrstDnwdHMI2LReq_Val/1 -> SeatMdSwtchArbtRunnable_sys/71(IfVeSMSbSecRwLtStLgrstDnwdHMI2LReq_Val_read)
  IfVeSMSbSecRwLtStLgrstInwdHMI2LReq_Val/1 -> SeatMdSwtchArbtRunnable_sys/72(IfVeSMSbSecRwLtStLgrstInwdHMI2LReq_Val_read)
  IfVeSMSbSecRwLtStLgrstOtwdHMI2LReq_Val/1 -> SeatMdSwtchArbtRunnable_sys/73(IfVeSMSbSecRwLtStLgrstOtwdHMI2LReq_Val_read)
  IfVeSMSbSecRwLtStLgrstUpwdHMI2LReq_Val/1 -> SeatMdSwtchArbtRunnable_sys/74(IfVeSMSbSecRwLtStLgrstUpwdHMI2LReq_Val_read)
  IfVeSMSbSecRwLtStLtwdHMI2LReq_Val/1 -> SeatMdSwtchArbtRunnable_sys/75(IfVeSMSbSecRwLtStLtwdHMI2LReq_Val_read)
  IfVeSMSbSecRwLtStRtwdHMI2LReq_Val/1 -> SeatMdSwtchArbtRunnable_sys/76(IfVeSMSbSecRwLtStRtwdHMI2LReq_Val_read)
  IfVeSMSbSecRwRtStArmScrnHMI2RReq_Val/1 -> SeatMdSwtchArbtRunnable_sys/77(IfVeSMSbSecRwRtStArmScrnHMI2RReq_Val_read)
  IfVeSMSbSecRwRtStBkReclnDnwdHMI2RReq_Val/1 -> SeatMdSwtchArbtRunnable_sys/78(IfVeSMSbSecRwRtStBkReclnDnwdHMI2RReq_Val_read)
  IfVeSMSbSecRwRtStBkReclnDnwdSwReq_Val/1 -> SeatMdSwtchArbtRunnable_sys/79(IfVeSMSbSecRwRtStBkReclnDnwdSwReq_Val_read)
  IfVeSMSbSecRwRtStBkReclnDnwdSwReqV_Val/1 -> SeatMdSwtchArbtRunnable_sys/80(IfVeSMSbSecRwRtStBkReclnDnwdSwReqV_Val_read)
  IfVeSMSbSecRwRtStBkReclnUpwdHMI2RReq_Val/1 -> SeatMdSwtchArbtRunnable_sys/81(IfVeSMSbSecRwRtStBkReclnUpwdHMI2RReq_Val_read)
  IfVeSMSbSecRwRtStBkReclnUpwdSwReq_Val/1 -> SeatMdSwtchArbtRunnable_sys/82(IfVeSMSbSecRwRtStBkReclnUpwdSwReq_Val_read)
  IfVeSMSbSecRwRtStBkReclnUpwdSwReqV_Val/1 -> SeatMdSwtchArbtRunnable_sys/83(IfVeSMSbSecRwRtStBkReclnUpwdSwReqV_Val_read)
  IfVeSMSbSecRwRtStBkwdHMI2RReq_Val/1 -> SeatMdSwtchArbtRunnable_sys/84(IfVeSMSbSecRwRtStBkwdHMI2RReq_Val_read)
  IfVeSMSbSecRwRtStBkwdSwReq_Val/1 -> SeatMdSwtchArbtRunnable_sys/85(IfVeSMSbSecRwRtStBkwdSwReq_Val_read)
  IfVeSMSbSecRwRtStBkwdSwReqV_Val/1 -> SeatMdSwtchArbtRunnable_sys/86(IfVeSMSbSecRwRtStBkwdSwReqV_Val_read)
  IfVeSMSbSecRwRtStFrwdHMI2RReq_Val/1 -> SeatMdSwtchArbtRunnable_sys/87(IfVeSMSbSecRwRtStFrwdHMI2RReq_Val_read)
  IfVeSMSbSecRwRtStFrwdSwReq_Val/1 -> SeatMdSwtchArbtRunnable_sys/88(IfVeSMSbSecRwRtStFrwdSwReq_Val_read)
  IfVeSMSbSecRwRtStFrwdSwReqV_Val/1 -> SeatMdSwtchArbtRunnable_sys/89(IfVeSMSbSecRwRtStFrwdSwReqV_Val_read)
  IfVeSMSbSecRwRtStFtDnwdHMI2RReq_Val/1 -> SeatMdSwtchArbtRunnable_sys/90(IfVeSMSbSecRwRtStFtDnwdHMI2RReq_Val_read)
  IfVeSMSbSecRwRtStFtUpwdHMI2RReq_Val/1 -> SeatMdSwtchArbtRunnable_sys/91(IfVeSMSbSecRwRtStFtUpwdHMI2RReq_Val_read)
  IfVeSMSbSecRwRtStHdrstBkwdHMI2RReq_Val/1 -> SeatMdSwtchArbtRunnable_sys/92(IfVeSMSbSecRwRtStHdrstBkwdHMI2RReq_Val_read)
  IfVeSMSbSecRwRtStHdrstDnwdHMI2RReq_Val/1 -> SeatMdSwtchArbtRunnable_sys/93(IfVeSMSbSecRwRtStHdrstDnwdHMI2RReq_Val_read)
  IfVeSMSbSecRwRtStHdrstFrwdHMI2RReq_Val/1 -> SeatMdSwtchArbtRunnable_sys/94(IfVeSMSbSecRwRtStHdrstFrwdHMI2RReq_Val_read)
  IfVeSMSbSecRwRtStHdrstUpwdHMI2RReq_Val/1 -> SeatMdSwtchArbtRunnable_sys/95(IfVeSMSbSecRwRtStHdrstUpwdHMI2RReq_Val_read)
  IfVeSMSbSecRwRtStLgrstDnwdHMI2RReq_Val/1 -> SeatMdSwtchArbtRunnable_sys/96(IfVeSMSbSecRwRtStLgrstDnwdHMI2RReq_Val_read)
  IfVeSMSbSecRwRtStLgrstDnwdSwReq_Val/1 -> SeatMdSwtchArbtRunnable_sys/97(IfVeSMSbSecRwRtStLgrstDnwdSwReq_Val_read)
  IfVeSMSbSecRwRtStLgrstDnwdSwReqV_Val/1 -> SeatMdSwtchArbtRunnable_sys/98(IfVeSMSbSecRwRtStLgrstDnwdSwReqV_Val_read)
  IfVeSMSbSecRwRtStLgrstInwdHMI2RReq_Val/1 -> SeatMdSwtchArbtRunnable_sys/99(IfVeSMSbSecRwRtStLgrstInwdHMI2RReq_Val_read)
  IfVeSMSbSecRwRtStLgrstOtwdHMI2RReq_Val/1 -> SeatMdSwtchArbtRunnable_sys/100(IfVeSMSbSecRwRtStLgrstOtwdHMI2RReq_Val_read)
  IfVeSMSbSecRwRtStLgrstUpwdHMI2RReq_Val/1 -> SeatMdSwtchArbtRunnable_sys/101(IfVeSMSbSecRwRtStLgrstUpwdHMI2RReq_Val_read)
  IfVeSMSbSecRwRtStLgrstUpwdSwReq_Val/1 -> SeatMdSwtchArbtRunnable_sys/102(IfVeSMSbSecRwRtStLgrstUpwdSwReq_Val_read)
  IfVeSMSbSecRwRtStLgrstUpwdSwReqV_Val/1 -> SeatMdSwtchArbtRunnable_sys/103(IfVeSMSbSecRwRtStLgrstUpwdSwReqV_Val_read)
  IfVeSMSbSecRwRtStLmbrHMI2RReq_Val/1 -> SeatMdSwtchArbtRunnable_sys/104(IfVeSMSbSecRwRtStLmbrHMI2RReq_Val_read)
  IfVeSMSbSecRwRtStLtwdHMI2RReq_Val/1 -> SeatMdSwtchArbtRunnable_sys/105(IfVeSMSbSecRwRtStLtwdHMI2RReq_Val_read)
  IfVeSMSbSecRwRtStRtwdHMI2RReq_Val/1 -> SeatMdSwtchArbtRunnable_sys/106(IfVeSMSbSecRwRtStRtwdHMI2RReq_Val_read)
  IfVeSMSbThdRLtStExpdSwReq_Val/1 -> SeatMdSwtchArbtRunnable_sys/107(IfVeSMSbThdRLtStExpdSwReq_Val_read)
  IfVeSMSbThdRLtStExpdSwReqV_Val/1 -> SeatMdSwtchArbtRunnable_sys/108(IfVeSMSbThdRLtStExpdSwReqV_Val_read)
  IfVeSMSbThdRRtStExpdSwReq_Val/1 -> SeatMdSwtchArbtRunnable_sys/109(IfVeSMSbThdRRtStExpdSwReq_Val_read)
  IfVeSMSbThdRRtStExpdSwReqV_Val/1 -> SeatMdSwtchArbtRunnable_sys/110(IfVeSMSbThdRRtStExpdSwReqV_Val_read)
  IfVeSMSbThdRwLtStBkReclnDnwdSwReq_Val/1 -> SeatMdSwtchArbtRunnable_sys/111(IfVeSMSbThdRwLtStBkReclnDnwdSwReq_Val_read)
  IfVeSMSbThdRwLtStBkReclnDnwdSwReqV_Val/1 -> SeatMdSwtchArbtRunnable_sys/112(IfVeSMSbThdRwLtStBkReclnDnwdSwReqV_Val_read)
  IfVeSMSbThdRwLtStBkReclnUpwdSwReq_Val/1 -> SeatMdSwtchArbtRunnable_sys/113(IfVeSMSbThdRwLtStBkReclnUpwdSwReq_Val_read)
  IfVeSMSbThdRwLtStBkReclnUpwdSwReqV_Val/1 -> SeatMdSwtchArbtRunnable_sys/114(IfVeSMSbThdRwLtStBkReclnUpwdSwReqV_Val_read)
  IfVeSMSbThdRwLtStBkwdSwReq_Val/1 -> SeatMdSwtchArbtRunnable_sys/115(IfVeSMSbThdRwLtStBkwdSwReq_Val_read)
  IfVeSMSbThdRwLtStBkwdSwReqV_Val/1 -> SeatMdSwtchArbtRunnable_sys/116(IfVeSMSbThdRwLtStBkwdSwReqV_Val_read)
  IfVeSMSbThdRwLtStFrwdSwReq_Val/1 -> SeatMdSwtchArbtRunnable_sys/117(IfVeSMSbThdRwLtStFrwdSwReq_Val_read)
  IfVeSMSbThdRwLtStFrwdSwReqV_Val/1 -> SeatMdSwtchArbtRunnable_sys/118(IfVeSMSbThdRwLtStFrwdSwReqV_Val_read)
  IfVeSMSbThdRwRtStBkReclnDnwdSwReq_Val/1 -> SeatMdSwtchArbtRunnable_sys/119(IfVeSMSbThdRwRtStBkReclnDnwdSwReq_Val_read)
  IfVeSMSbThdRwRtStBkReclnDnwdSwReqV_Val/1 -> SeatMdSwtchArbtRunnable_sys/120(IfVeSMSbThdRwRtStBkReclnDnwdSwReqV_Val_read)
  IfVeSMSbThdRwRtStBkReclnUpwdSwReq_Val/1 -> SeatMdSwtchArbtRunnable_sys/121(IfVeSMSbThdRwRtStBkReclnUpwdSwReq_Val_read)
  IfVeSMSbThdRwRtStBkReclnUpwdSwReqV_Val/1 -> SeatMdSwtchArbtRunnable_sys/122(IfVeSMSbThdRwRtStBkReclnUpwdSwReqV_Val_read)
  IfVeSMSbThdRwRtStBkwdSwReq_Val/1 -> SeatMdSwtchArbtRunnable_sys/123(IfVeSMSbThdRwRtStBkwdSwReq_Val_read)
  IfVeSMSbThdRwRtStBkwdSwReqV_Val/1 -> SeatMdSwtchArbtRunnable_sys/124(IfVeSMSbThdRwRtStBkwdSwReqV_Val_read)
  IfVeSMSbThdRwRtStFrwdSwReq_Val/1 -> SeatMdSwtchArbtRunnable_sys/125(IfVeSMSbThdRwRtStFrwdSwReq_Val_read)
  IfVeSMSbThdRwRtStFrwdSwReqV_Val/1 -> SeatMdSwtchArbtRunnable_sys/126(IfVeSMSbThdRwRtStFrwdSwReqV_Val_read)
  IfVeSMSeSecLTMemHMI2LReq1_Val/1 -> SeatMdSwtchArbtRunnable_sys/127(IfVeSMSeSecLTMemHMI2LReq1_Val_read)
  IfVeSMSeSecLTMemHMI2RReq1_Val/1 -> SeatMdSwtchArbtRunnable_sys/128(IfVeSMSeSecLTMemHMI2RReq1_Val_read)
  IfVeSMSuSeatPosEnable_Val/1 -> SeatMdSwtchArbtRunnable_sys/129(IfVeSMSuSeatPosEnable_Val_read)
  StSlctSwReq_Val/1 -> SeatMdSwtchArbtRunnable_sys/130(StSlctSwReq_Val_read)
  StSlctSwReqV_Val/1 -> SeatMdSwtchArbtRunnable_sys/131(StSlctSwReqV_Val_read)
  SeatMdSwtchArbtRunnable_sys/1(IfVeSMSbIs2LStSwAct_Val_write) -> IfVeSMSbIs2LStSwAct_Val/1
  SeatMdSwtchArbtRunnable_sys/2(IfVeSMSbIs2RStSwAct_Val_write) -> IfVeSMSbIs2RStSwAct_Val/1
  SeatMdSwtchArbtRunnable_sys/3(IfVeSMSbIs3LStSwAct_Val_write) -> IfVeSMSbIs3LStSwAct_Val/1
  SeatMdSwtchArbtRunnable_sys/4(IfVeSMSbIs3RStSwAct_Val_write) -> IfVeSMSbIs3RStSwAct_Val/1
  SeatMdSwtchArbtRunnable_sys/5(IfVeSMSbIsDrvStSwAct_Val_write) -> IfVeSMSbIsDrvStSwAct_Val/1
  SeatMdSwtchArbtRunnable_sys/6(IfVeSMSbIsPasStSwAct_Val_write) -> IfVeSMSbIsPasStSwAct_Val/1
  SeatMdSwtchArbtRunnable/1 -> SeatMdSwtchArbtRunnable_sys/Trigger
  IfVeSMSuRrLtStFtUpwdPstnHMI2LReq_Val/1 -> SeatMdSwtchArbtRunnable_sys/132(IfVeSMSuRrLtStFtUpwdPstnHMI2LReq_Val_read)
  IfVeSMSuRrLtStFtUpwdPstnHMI2LReqV_Val/1 -> SeatMdSwtchArbtRunnable_sys/133(IfVeSMSuRrLtStFtUpwdPstnHMI2LReqV_Val_read)
  IfVeSMSuRrRtStFtUpwdPstnHMI2RReq_Val/1 -> SeatMdSwtchArbtRunnable_sys/134(IfVeSMSuRrRtStFtUpwdPstnHMI2RReq_Val_read)
  IfVeSMSuRrRtStFtUpwdPstnHMI2RReqV_Val/1 -> SeatMdSwtchArbtRunnable_sys/135(IfVeSMSuRrRtStFtUpwdPstnHMI2RReqV_Val_read)
  IfVeSMSbSecRwLtStFtClsHMI2LReq_Val/1 -> SeatMdSwtchArbtRunnable_sys/136(IfVeSMSbSecRwLtStFtClsHMI2LReq_Val_read)
  IfVeSMSbSecRwLtStFtOpenHMI2LReq_Val/1 -> SeatMdSwtchArbtRunnable_sys/137(IfVeSMSbSecRwLtStFtOpenHMI2LReq_Val_read)
  IfVeSMSbSecRwRtStFtClsHMI2LReq_Val/1 -> SeatMdSwtchArbtRunnable_sys/138(IfVeSMSbSecRwRtStFtClsHMI2LReq_Val_read)
  IfVeSMSbSecRwRtStFtOpenHMI2LReq_Val/1 -> SeatMdSwtchArbtRunnable_sys/139(IfVeSMSbSecRwRtStFtOpenHMI2LReq_Val_read)
  IfSecRwLtStCushnFrtDnwdHMI2LReq_Val/1 -> SeatMdSwtchArbtRunnable_sys/140(IfSecRwLtStCushnFrtDnwdHMI2LReq_Val_read)
  IfSecRwLtStCushnFrtUpwdDnwdMovmtVirtCtrlReq_Val/1 -> SeatMdSwtchArbtRunnable_sys/141(IfSecRwLtStCushnFrtUpwdDnwdMovmtVirtCtrlReq_Val_read)
  IfSecRwLtStCushnFrtUpwdHMI2LReq_Val/1 -> SeatMdSwtchArbtRunnable_sys/142(IfSecRwLtStCushnFrtUpwdHMI2LReq_Val_read)
  IfSecRwLtStFwdBkwdMovmtVirtCtrlReq_Val/1 -> SeatMdSwtchArbtRunnable_sys/143(IfSecRwLtStFwdBkwdMovmtVirtCtrlReq_Val_read)
  IfSecRwLtStLgrstOtwdInwdMovmtVirtCtrlReq_Val/1 -> SeatMdSwtchArbtRunnable_sys/144(IfSecRwLtStLgrstOtwdInwdMovmtVirtCtrlReq_Val_read)
  IfSecRwLtStLgrstUpwdDnwdMovmtVirtCtrlReq_Val/1 -> SeatMdSwtchArbtRunnable_sys/145(IfSecRwLtStLgrstUpwdDnwdMovmtVirtCtrlReq_Val_read)
  IfSecRwLtStRclUpwdDnwdMovmtVirtCtrlReq_Val/1 -> SeatMdSwtchArbtRunnable_sys/146(IfSecRwLtStRclUpwdDnwdMovmtVirtCtrlReq_Val_read)
  IfSecRwRtStCushnFrtDnwdHMI2LReq_Val/1 -> SeatMdSwtchArbtRunnable_sys/147(IfSecRwRtStCushnFrtDnwdHMI2LReq_Val_read)
  IfSecRwRtStCushnFrtUpwdDnwdMovmtVirtCtrlReq_Val/1 -> SeatMdSwtchArbtRunnable_sys/148(IfSecRwRtStCushnFrtUpwdDnwdMovmtVirtCtrlReq_Val_read)
  IfSecRwRtStCushnFrtUpwdHMI2LReq_Val/1 -> SeatMdSwtchArbtRunnable_sys/149(IfSecRwRtStCushnFrtUpwdHMI2LReq_Val_read)
  IfSecRwRtStFwdBkwdMovmtVirtCtrlReq_Val/1 -> SeatMdSwtchArbtRunnable_sys/150(IfSecRwRtStFwdBkwdMovmtVirtCtrlReq_Val_read)
  IfSecRwRtStLgrstOtwdInwdMovmtVirtCtrlReq_Val/1 -> SeatMdSwtchArbtRunnable_sys/151(IfSecRwRtStLgrstOtwdInwdMovmtVirtCtrlReq_Val_read)
  IfSecRwRtStLgrstUpwdDnwdMovmtVirtCtrlReq_Val/1 -> SeatMdSwtchArbtRunnable_sys/152(IfSecRwRtStLgrstUpwdDnwdMovmtVirtCtrlReq_Val_read)
  IfSecRwRtStRclUpwdDnwdMovmtVirtCtrlReq_Val/1 -> SeatMdSwtchArbtRunnable_sys/153(IfSecRwRtStRclUpwdDnwdMovmtVirtCtrlReq_Val_read)
  IfSecRwRtStLgrstInwdSwReq_Val/1 -> SeatMdSwtchArbtRunnable_sys/154(IfSecRwRtStLgrstInwdSwReq_Val_read)
  IfSecRwRtStLgrstInwdSwReqV_Val/1 -> SeatMdSwtchArbtRunnable_sys/155(IfSecRwRtStLgrstInwdSwReqV_Val_read)
  IfSecRwRtStLgrstOtwdSwReq_Val/1 -> SeatMdSwtchArbtRunnable_sys/156(IfSecRwRtStLgrstOtwdSwReq_Val_read)
  IfSecRwRtStLgrstOtwdSwReqV_Val/1 -> SeatMdSwtchArbtRunnable_sys/157(IfSecRwRtStLgrstOtwdSwReqV_Val_read)
  IfVeSMSbPassStBkReclnDnwdMovBosSwAct_Val/1 -> SeatMdSwtchArbtRunnable_sys/158(IfVeSMSbPassStBkReclnDnwdMovBosSwAct_Val_read)
  IfVeSMSbPassStBkReclnDnwdMovBosSwActV_Val/1 -> SeatMdSwtchArbtRunnable_sys/159(IfVeSMSbPassStBkReclnDnwdMovBosSwActV_Val_read)
  IfVeSMSbPassStBkReclnUpwdMovBosSwAct_Val/1 -> SeatMdSwtchArbtRunnable_sys/160(IfVeSMSbPassStBkReclnUpwdMovBosSwAct_Val_read)
  IfVeSMSbPassStBkReclnUpwdMovBosSwActV_Val/1 -> SeatMdSwtchArbtRunnable_sys/161(IfVeSMSbPassStBkReclnUpwdMovBosSwActV_Val_read)
  IfVeSMSbPassStBkwdMovBosSwAct_Val/1 -> SeatMdSwtchArbtRunnable_sys/162(IfVeSMSbPassStBkwdMovBosSwAct_Val_read)
  IfVeSMSbPassStBkwdMovBosSwActV_Val/1 -> SeatMdSwtchArbtRunnable_sys/163(IfVeSMSbPassStBkwdMovBosSwActV_Val_read)
  IfVeSMSbPassStFrwdMovBosSwAct_Val/1 -> SeatMdSwtchArbtRunnable_sys/164(IfVeSMSbPassStFrwdMovBosSwAct_Val_read)
  IfVeSMSbPassStFrwdMovBosSwActV_Val/1 -> SeatMdSwtchArbtRunnable_sys/165(IfVeSMSbPassStFrwdMovBosSwActV_Val_read)
  IfSecRwRtStZeroGrvyDnwdSwReq_Val/1 -> SeatMdSwtchArbtRunnable_sys/166(IfSecRwRtStZeroGrvyDnwdSwReq_Val_read)
  IfSecRwRtStZeroGrvyDnwdSwReqV_Val/1 -> SeatMdSwtchArbtRunnable_sys/167(IfSecRwRtStZeroGrvyDnwdSwReqV_Val_read)
  IfSecRwRtStZeroGrvyUpwdSwReq_Val/1 -> SeatMdSwtchArbtRunnable_sys/168(IfSecRwRtStZeroGrvyUpwdSwReq_Val_read)
  IfSecRwRtStZeroGrvyUpwdSwReqV_Val/1 -> SeatMdSwtchArbtRunnable_sys/169(IfSecRwRtStZeroGrvyUpwdSwReqV_Val_read)
  SecRwRtStBkReclnDnwdMovBossSwReq_Val/1 -> SeatMdSwtchArbtRunnable_sys/170(SecRwRtStBkReclnDnwdMovBossSwReq_Val_read)
  SecRwRtStBkReclnDnwdMovBossSwReqV_Val/1 -> SeatMdSwtchArbtRunnable_sys/171(SecRwRtStBkReclnDnwdMovBossSwReqV_Val_read)
  SecRwRtStBkReclnUpwdMovBossSwReq_Val/1 -> SeatMdSwtchArbtRunnable_sys/172(SecRwRtStBkReclnUpwdMovBossSwReq_Val_read)
  SecRwRtStBkReclnUpwdMovBossSwReqV_Val/1 -> SeatMdSwtchArbtRunnable_sys/173(SecRwRtStBkReclnUpwdMovBossSwReqV_Val_read)
  SecRwRtStBkwdMovBossSwReq_Val/1 -> SeatMdSwtchArbtRunnable_sys/174(SecRwRtStBkwdMovBossSwReq_Val_read)
  SecRwRtStBkwdMovBossSwReqV_Val/1 -> SeatMdSwtchArbtRunnable_sys/175(SecRwRtStBkwdMovBossSwReqV_Val_read)
  SecRwRtStFrwdMovBossSwReq_Val/1 -> SeatMdSwtchArbtRunnable_sys/176(SecRwRtStFrwdMovBossSwReq_Val_read)
  SecRwRtStFrwdMovBossSwReqV_Val/1 -> SeatMdSwtchArbtRunnable_sys/177(SecRwRtStFrwdMovBossSwReqV_Val_read)
  PassStPosRclRspStat_Val/1 -> SeatMdSwtchArbtRunnable_sys/178(PassStPosRclRspStat_Val_read)
